simulink model "FullHopper_k"  (R2020a)
settings: Solver=ode4  StartTime=0.0  StopTime=7.5  FixedStep=0.0005  RelTol=1e-3
model workspace (MAT data in the model file):
  Mass = 35
  T_stim = 0.4
  amplitude = 1
  k_shoe = 20000
  thickness = 0.025
undefined symbols (not defined in the file): dpMass0
settings Model: OrderedModelArguments=off  Creator=jmei13  LastModifiedBy=jmei13
settings DebuggingCC: AlgebraicLoopMsg=none  ArtificialAlgebraicLoopMsg=none  UnconnectedInputMsg=none  UnconnectedOutputMsg=none  UnconnectedLineMsg=none

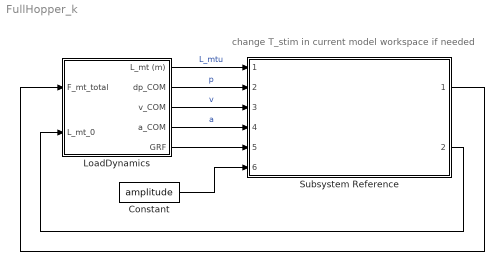
== system FullHopper_k ==
  note: change T_stim in current model workspace if needed
  Constant : Constant  Value=amplitude
  LoadDynamics : Subsystem
  Subsystem Reference : Subsystem  ReferencedSubsystem=muscle_dynamics_subsystem
  wires:
  LoadDynamics/1(L_mt (m)) -> Subsystem Reference/1  "L_mtu"
  LoadDynamics/2(dp_COM) -> Subsystem Reference/2  "p"
  LoadDynamics/3(v_COM) -> Subsystem Reference/3  "v"
  LoadDynamics/5(GRF) -> Subsystem Reference/5
  Constant/1 -> Subsystem Reference/6
  Subsystem Reference/1 -> LoadDynamics/1(F_mt_total)
  Subsystem Reference/2 -> LoadDynamics/2(L_mt_0)
  LoadDynamics/4(a_COM) -> Subsystem Reference/4  "a"

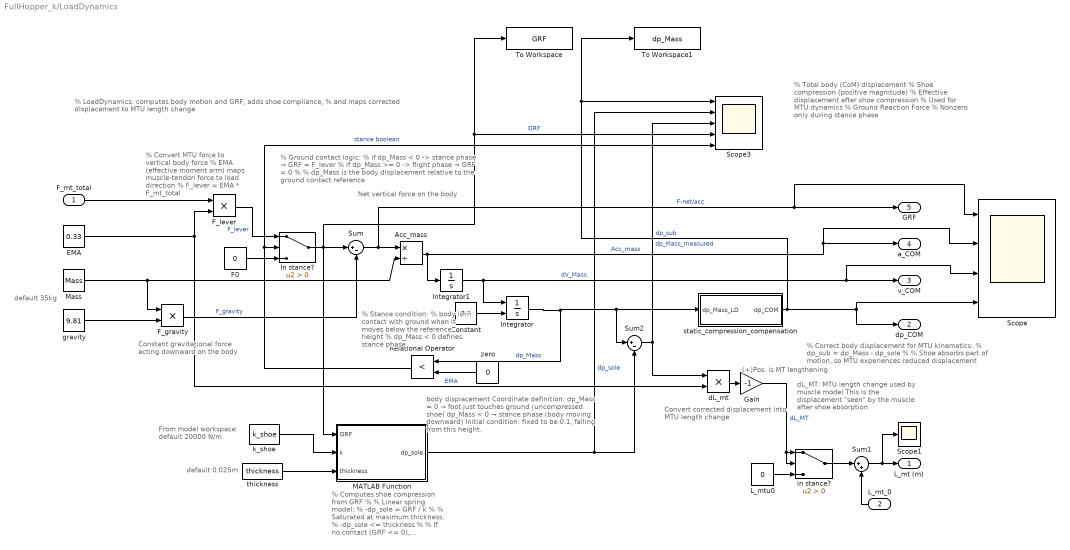
== system FullHopper_k/LoadDynamics ==
  note: % Total body (CoM) displacement
      |
      | % Shoe compression (positive magnitude)
      |
      | % Effective displacement after shoe compression
      | % Used for MTU dynamics
      |
      | % Ground Reaction Force
      | % Nonzero only during stance phase
  note: % LoadDynamics: computes body motion and GRF, adds shoe compliance,
      | % and maps corrected displacement to MTU length change
  note: dL_MT:
      | MTU length change used by muscle model
      | This is the displacement "seen" by the muscle after shoe absorption
  note: Convert corrected displacement into MTU length change
  note: % Correct body displacement for MTU kinematics:
      | % dp_sub = dp_Mass - dp_sole
      | %
      | % Shoe absorbs part of motion, so MTU experiences reduced displacement
  note: % Computes shoe compression from GRF
      | %
      | % Linear spring model:
      | % -dp_sole = GRF / k
      | %
      | % Saturated at maximum thickness:
      | % -dp_sole <= thickness
      | %
      | % If no contact (GRF <= 0), compression = 0
  note: body displacement
      | Coordinate definition:
      | dp_Mass = 0 → foot just touches ground (uncompressed shoe)
      | dp_Mass < 0 → stance phase (body moving downward)
      |
      | Initial condition: fixed to be 0.1, falling from this height.
  note: Net vertical force on the body
  note: % Stance condition:
      | % body is in contact with ground when it moves below the reference height
      | % dp_Mass < 0 defines stance phase
  note: % Ground contact logic:
      | % if dp_Mass < 0 -> stance phase → GRF = F_lever
      | % if dp_Mass >= 0 -> flight phase → GRF = 0
      | %
      | % dp_Mass is the body displacement relative to the ground contact reference
  note: Constant gravitational force acting downward on the body
  note: From model workspace:
      | default 20000 N/m
  note: (+)Pos. is MT
      | lengthening
  note: default 0.025m
  note: % Convert MTU force to vertical body force
      | % EMA (effective moment arm) maps muscle-tendon force to load direction
      | % F_lever = EMA * F_mt_total
  note: default 35kg
  F_mt_total : Inport
  L_mt_0 : Inport  Port=2
  Acc_mass : Product  Inputs=*/
  Constant : Constant  Value=0.1
  EMA : Constant  Value=0.33
  F0 : Constant  Value=0
  F_gravity : Product  RndMeth=Zero
  F_lever : Product  RndMeth=Zero
  Gain : Gain  Gain=-1
  In stance? : Switch  Criteria=u2 > Threshold
  Integrator : Integrator  InitialConditionSource=external  InitialCondition=dpMass0
  Integrator1 : Integrator
  L_mtu0 : Constant  Value=0
  MATLAB Function : MATLAB Function  TreatAsAtomicUnit=on
  Mass : Constant  Value=Mass
  Relational Operator : RelationalOperator  Operator=<  OutDataTypeStr=boolean  RndMeth=Simplest
  Scope : Scope  NumInputPorts=4
  Scope1 : Scope
  Scope3 : Scope  NumInputPorts=5
  Sum : Sum  Inputs=|+-
  Sum1 : Sum  Inputs=|++
  Sum2 : Sum  Inputs=|+-
  To Workspace : ToWorkspace  VariableName=GRF  SaveFormat=Timeseries  SampleTime=-1
  To Workspace1 : ToWorkspace  VariableName=dp_Mass  SaveFormat=Timeseries  SampleTime=-1
  dL_mt : Product  RndMeth=Zero
  gravity : Constant  Value=9.81
  "in stance? " : Switch  Criteria=u2 > Threshold
  k_shoe : Constant  Value=k_shoe
  static_compression_compensation : Subsystem
  thickness : Constant  Value=thickness
  zero : Constant  Value=0
  L_mt (m) : Outport
  dp_COM : Outport  Port=2
  v_COM : Outport  Port=3
  a_COM : Outport  Port=4
  GRF : Outport  Port=5
  wires:
  Integrator1/1 -> Integrator/1, Scope/3, v_COM/1  "dV_Mass"
  Sum1/1 -> Scope1/1, L_mt (m)/1
  L_mt_0/1 -> Sum1/2
  Acc_mass/1 -> Scope/2, a_COM/1, Integrator1/1  "Acc_mass"
  F0/1 -> In stance?/3
  Sum/1 -> Scope/1, GRF/1, Acc_mass/1  "F-net/acc"
  F_mt_total/1 -> F_lever/1
  Gain/1 -> "in stance? "/1, "in stance? "/2  "dL_MT"
  dL_mt/1 -> Gain/1
  F_lever/1 -> In stance?/1  "F_lever"
  Integrator/1 -> Relational Operator/1, Sum2/1, static_compression_compensation/1(dp_Mass_LD)  "dp_Mass"
  F_gravity/1 -> Sum/2  "F_gravity"
  EMA/1 -> F_lever/2, dL_mt/2  "EMA"
  gravity/1 -> F_gravity/2
  Mass/1 -> F_gravity/1, Acc_mass/2
  L_mtu0/1 -> "in stance? "/3
  In stance?/1 -> Sum/1, To Workspace/1, Scope3/4, MATLAB Function/1(GRF)  "GRF"
  "in stance? "/1 -> Sum1/1
  MATLAB Function/1(dp_sole) -> Scope3/2, Sum2/2  "dp_sole"
  Sum2/1 -> Scope3/3, dL_mt/1  "dp_sub"
  zero/1 -> Relational Operator/2
  Relational Operator/1 -> In stance?/2, Scope3/5  "stance boolean"
  k_shoe/1 -> MATLAB Function/2(k)
  thickness/1 -> MATLAB Function/3(thickness)
  Constant/1 -> Integrator/2
  static_compression_compensation/1(dp_COM) -> Scope/4, dp_COM/1, To Workspace1/1, Scope3/1  "dp_Mass_measured"

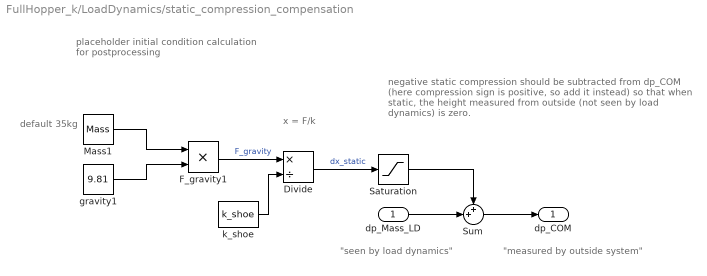
== system FullHopper_k/LoadDynamics/static_compression_compensation ==
  note: x = F/k
  note: placeholder initial condition calculation
      | for postprocessing
  note: default 35kg
  note: negative static compression should be subtracted from dp_COM
      | (here compression sign is positive, so add it instead)
      | so that when static, the height measured from outside
      | (not seen by load dynamics) is zero.
  note: "seen by load dynamics"
  note: "measured by outside system"
  dp_Mass_LD : Inport
  Divide : Product  Inputs=*/
  F_gravity1 : Product  RndMeth=Zero
  Mass1 : Constant  Value=Mass
  Saturation : Saturate  UpperLimit=thickness  LowerLimit=0
  Sum : Sum  Inputs=++|
  gravity1 : Constant  Value=9.81
  k_shoe : Constant  Value=k_shoe
  dp_COM : Outport
  wires:
  F_gravity1/1 -> Divide/1  "F_gravity"
  Saturation/1 -> Sum/1
  gravity1/1 -> F_gravity1/2
  Divide/1 -> Saturation/1  "dx_static"
  Mass1/1 -> F_gravity1/1
  Sum/1 -> dp_COM/1
  dp_Mass_LD/1 -> Sum/2
  k_shoe/1 -> Divide/2

== matlab function FullHopper_k/LoadDynamics/MATLAB Function ==
  data: GRF input; dp_sole output; k input; thickness input
function dp_sole = shoe_disp(GRF,k,thickness)
% Computes shoe (sole) compression based on ground reaction force (GRF)
% This compression is subtracted from CoM displacement:
%   dp_sub = dp_Mass - dp_sole
% Inputs:
%   GRF       - Ground Reaction Force (N)
%   k         - Shoe stiffness (N/m)
%   thickness - Maximum allowable compression of the sole (m)
%
% Output:
%   dp_sole   - Displacement/Compression of the shoe sole (m, negative value)
%   taken as negative to match the displacement coordinates like dp_COM.

% Case 1: No contact (flight phase)
% If GRF is zero or negative, the foot is not in contact with the ground
% → no compression in the shoe
if GRF <= 0
    dp_sole = 0;

else
    % Case 2: Foot is in contact (stance phase)
    
    % Compute linear spring compression using Hooke's Law:
    %   F = kx  →  x = F/k
    x = GRF / k;
    
    % Limit compression to the physical thickness of the sole
    % This prevents unrealistic "over-compression"
    if x > thickness
        x = thickness;
    end
    
    % Output compression
    % Note: dp_sole is defined as a positive quantity (magnitude of compression)
    dp_sole = x;
end

% reflect the sign to match displacement convention: 
% upwards is positive

dp_sole = -dp_sole;
